simulink subsystem "Vehicle_Forces_Moments"  (R2025b)
settings: Solver=VariableStepAuto  StartTime=0.0  StopTime=10.0  RelTol=1e-3
libraries: aerolibactuator x2
settings Model: Creator=cdriggs  LastModifiedBy=cdriggs

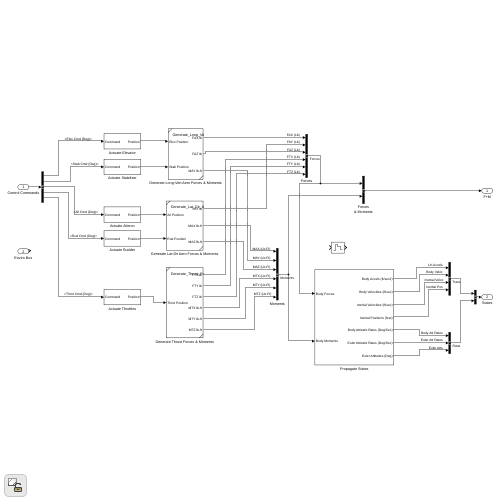
[thumbnail: Simulink's stored preview of the top-level diagram]
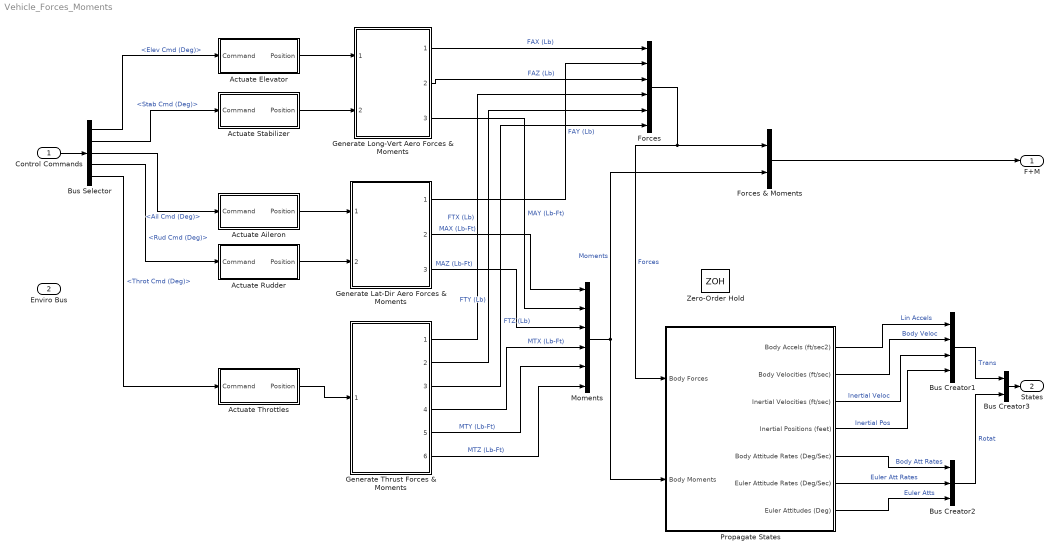
== system Vehicle_Forces_Moments ==
  Control Commands : Inport
  Enviro Bus : Inport  Port=2
  Actuate Aileron : Subsystem
  Actuate Elevator : Subsystem
  Actuate Rudder : Subsystem
  Actuate Stabilizer : Subsystem
  Actuate Throttles : Subsystem
  Bus Creator1 : BusCreator  Inputs=4
  Bus Creator2 : BusCreator  Inputs=3
  Bus Creator3 : BusCreator  Inputs=2
  Bus Selector : BusSelector  OutputSignals=Elev Cmd (Deg),Stab Cmd (Deg),Ail Cmd (Deg),Rud Cmd (Deg),Throt Cmd (Deg)
  Forces : BusCreator  Inputs=6
  Forces & Moments : BusCreator  Inputs=2
  Generate Lat-Dir Aero Forces & Moments : Subsystem  ReferencedSubsystem=Lat_Dir_Aero_Forces_Moments
  Generate Long-Vert Aero Forces & Moments : Subsystem  ReferencedSubsystem=Long_Vert_Aero_Forces_Moments
  Generate Thrust Forces & Moments : Subsystem  ReferencedSubsystem=Thrust_Forces_Moments
  Moments : BusCreator  Inputs=6
  Propagate States : Subsystem
  Zero-Order Hold : ZeroOrderHold  SampleTime=-1
  F+M : Outport
  States : Outport  Port=2
  wires:
  Forces & Moments/1 -> F+M/1
  Bus Creator1/1 -> Bus Creator3/1  "Trans"
  Bus Creator2/1 -> Bus Creator3/2  "Rotat"
  Bus Creator3/1 -> States/1
  Propagate States/1(Body Accels (ft/sec2)) -> Bus Creator1/1  "Lin Accels"
  Propagate States/2(Body Velocities (ft/sec)) -> Bus Creator1/2  "Body Veloc"
  Propagate States/3(Inertial Velocities (ft/sec)) -> Bus Creator1/3  "Inertial Veloc"
  Propagate States/4(Inertial Positions (feet)) -> Bus Creator1/4  "Inertial Pos"
  Propagate States/5(Body Attitude Rates (Deg/Sec)) -> Bus Creator2/1  "Body Att Rates"
  Propagate States/6(Euler Attitude Rates (Deg/Sec)) -> Bus Creator2/2  "Euler Att Rates"
  Propagate States/7(Euler Attitudes (Deg)) -> Bus Creator2/3  "Euler Atts"
  Generate Long-Vert Aero Forces & Moments/1 -> Forces/1  "FAX (Lb)"
  Generate Long-Vert Aero Forces & Moments/2 -> Forces/3  "FAZ (Lb)"
  Generate Lat-Dir Aero Forces & Moments/1 -> Forces/2  "FAY (Lb)"
  Generate Lat-Dir Aero Forces & Moments/2 -> Moments/1  "MAX (Lb-Ft)"
  Generate Long-Vert Aero Forces & Moments/3 -> Moments/2  "MAY (Lb-Ft)"
  Generate Lat-Dir Aero Forces & Moments/3 -> Moments/3  "MAZ (Lb-Ft)"
  Forces/1 -> Forces & Moments/1, Propagate States/1(Body Forces)  "Forces"
  Moments/1 -> Propagate States/2(Body Moments), Forces & Moments/2  "Moments"
  Control Commands/1 -> Bus Selector/1
  Bus Selector/1 -> Actuate Elevator/1(Command)  "<Elev Cmd (Deg)>"
  Actuate Elevator/1(Position) -> Generate Long-Vert Aero Forces & Moments/1
  Actuate Aileron/1(Position) -> Generate Lat-Dir Aero Forces & Moments/1
  Actuate Rudder/1(Position) -> Generate Lat-Dir Aero Forces & Moments/2
  Bus Selector/4 -> Actuate Rudder/1(Command)  "<Rud Cmd (Deg)>"
  Bus Selector/3 -> Actuate Aileron/1(Command)  "<Ail Cmd (Deg)>"
  Actuate Throttles/1(Position) -> Generate Thrust Forces & Moments/1
  Bus Selector/5 -> Actuate Throttles/1(Command)  "<Throt Cmd (Deg)>"
  Bus Selector/2 -> Actuate Stabilizer/1(Command)  "<Stab Cmd (Deg)>"
  Actuate Stabilizer/1(Position) -> Generate Long-Vert Aero Forces & Moments/2
  Generate Thrust Forces & Moments/1 -> Forces/4  "FTX (Lb)"
  Generate Thrust Forces & Moments/2 -> Forces/5  "FTY (Lb)"
  Generate Thrust Forces & Moments/3 -> Forces/6  "FTZ (Lb)"
  Generate Thrust Forces & Moments/4 -> Moments/4  "MTX (Lb-Ft)"
  Generate Thrust Forces & Moments/5 -> Moments/5  "MTY (Lb-Ft)"
  Generate Thrust Forces & Moments/6 -> Moments/6  "MTZ (Lb-Ft)"

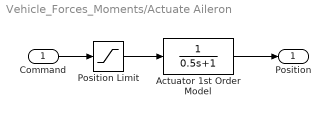
== system Vehicle_Forces_Moments/Actuate Aileron ==
  Command : Inport
  Actuator 1st Order Model : TransferFcn  Denominator=[0.5 1]
  Position Limit : Saturate  UpperLimit=30  LowerLimit=-30
  Position : Outport
  wires:
  Actuator 1st Order Model/1 -> Position/1
  Position Limit/1 -> Actuator 1st Order Model/1
  Command/1 -> Position Limit/1

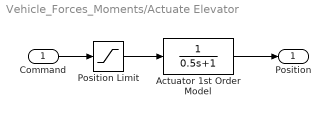
== system Vehicle_Forces_Moments/Actuate Elevator ==
  Command : Inport
  Actuator 1st Order Model : TransferFcn  Denominator=[0.5 1]
  Position Limit : Saturate  UpperLimit=30  LowerLimit=-30
  Position : Outport
  wires:
  Actuator 1st Order Model/1 -> Position/1
  Position Limit/1 -> Actuator 1st Order Model/1
  Command/1 -> Position Limit/1

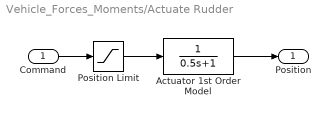
== system Vehicle_Forces_Moments/Actuate Rudder ==
  Command : Inport
  Actuator 1st Order Model : TransferFcn  Denominator=[0.5 1]
  Position Limit : Saturate  UpperLimit=30  LowerLimit=-30
  Position : Outport
  wires:
  Actuator 1st Order Model/1 -> Position/1
  Position Limit/1 -> Actuator 1st Order Model/1
  Command/1 -> Position Limit/1

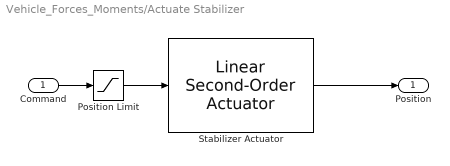
== system Vehicle_Forces_Moments/Actuate Stabilizer ==
  Command : Inport
  Position Limit : Saturate  UpperLimit=15  LowerLimit=-5
  Stabilizer Actuator : aerolibactuator/Linear Second-Order Actuator  wn_fin=0.3  z_fin=1.0  fin_act_0=0  fin_act_vel=0
  Position : Outport
  wires:
  Stabilizer Actuator/1 -> Position/1
  Position Limit/1 -> Stabilizer Actuator/1
  Command/1 -> Position Limit/1

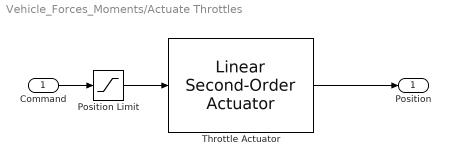
== system Vehicle_Forces_Moments/Actuate Throttles ==
  Command : Inport
  Position Limit : Saturate  UpperLimit=100  LowerLimit=0
  Throttle Actuator : aerolibactuator/Linear Second-Order Actuator  wn_fin=1  z_fin=1.0  fin_act_0=0  fin_act_vel=0
  Position : Outport
  wires:
  Throttle Actuator/1 -> Position/1
  Position Limit/1 -> Throttle Actuator/1
  Command/1 -> Position Limit/1

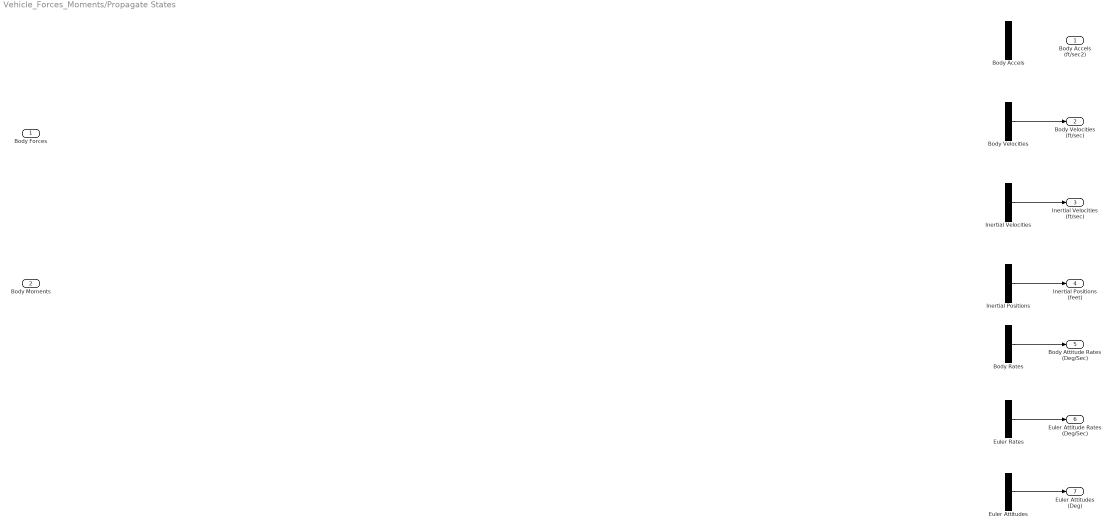
== system Vehicle_Forces_Moments/Propagate States ==
  Body Forces : Inport
  Body Moments : Inport  Port=2
  Body Accels : BusCreator  Inputs=3
  Body Rates : BusCreator  Inputs=3
  Body Velocities : BusCreator  Inputs=3
  Euler Attitudes : BusCreator  Inputs=3
  Euler Rates : BusCreator  Inputs=3
  Inertial Positions : BusCreator  Inputs=3
  Inertial Velocities : BusCreator  Inputs=3
  Body Accels (ft/sec2) : Outport
  Body Velocities (ft/sec) : Outport  Port=2
  Inertial Velocities (ft/sec) : Outport  Port=3
  Inertial Positions (feet) : Outport  Port=4
  Body Attitude Rates (Deg/Sec) : Outport  Port=5
  Euler Attitude Rates (Deg/Sec) : Outport  Port=6
  Euler Attitudes (Deg) : Outport  Port=7
  wires:
  ? -> Body Velocities/2  "v (Feet/Sec)"
  ? -> Body Velocities/1  "u (Feet/Sec)"
  ? -> Body Velocities/3  "w (Feet/Sec)"
  ? -> Inertial Velocities/2  "East-West Velocity (Feet/Sec)"
  ? -> Inertial Velocities/1  "North-South Velocity (Feet/Sec)"
  ? -> Inertial Velocities/3  "Inertial Vertical Speed (Feet/Sec)"
  ? -> Inertial Positions/2  "Longitude (Feet)"
  ? -> Inertial Positions/1  "Latitude (Feet)"
  ? -> Inertial Positions/3  "Inertial Altitude (Feet)"
  ? -> Body Rates/2  "Roll Rate (Deg/Sec)"
  ? -> Body Rates/3  "Yaw Rate (Deg/Sec)"
  ? -> Body Rates/1  "Pitch Rate (Deg/Sec)"
  ? -> Euler Rates/2  "Roll Att Rate (Deg/Sec)"
  ? -> Euler Rates/3  "Heading Att Rate (Deg/Sec)"
  ? -> Euler Rates/1  "Pitch Att Rate (Deg/Sec)"
  ? -> Body Accels/3  "Vertical Accel (Ft/Sec^2)"
  ? -> Body Accels/2  "Lateral Accel (Ft/Sec^2)"
  ? -> Body Accels/1  "Longitudinal Accel (Ft/Sec^2)"
  Body Velocities/1 -> Body Velocities (ft/sec)/1
  Inertial Velocities/1 -> Inertial Velocities (ft/sec)/1
  Inertial Positions/1 -> Inertial Positions (feet)/1
  Body Rates/1 -> Body Attitude Rates (Deg/Sec)/1
  Euler Rates/1 -> Euler Attitude Rates (Deg/Sec)/1
  ? -> Euler Attitudes/1  "Pitch Attitude (Deg)"
  ? -> Euler Attitudes/2  "Roll Attitude (Deg)"
  ? -> Euler Attitudes/3  "Heading (Deg)"
  Euler Attitudes/1 -> Euler Attitudes (Deg)/1
